simulink model "actuatorsTestHarness"  (R2024a)
settings: configuration reference "standardSILConfiguraitonParams" (kept outside this file)
undefined symbols (not defined in the file): aileronDeflRateLimit_degps, elevatorDeflRateLimit_degps, maxAilDefl_deg, maxElevatorDefl_deg, maxRudderDefl_deg, rudderDeflRateLimit_degps, stepSize_s
settings Model: SimulationMode=accelerator  Creator=jerem  LastModifiedBy=jerem
settings ConfigSetRef: SourceName=standardSILConfiguraitonParams  SourceLocation=Base Workspace

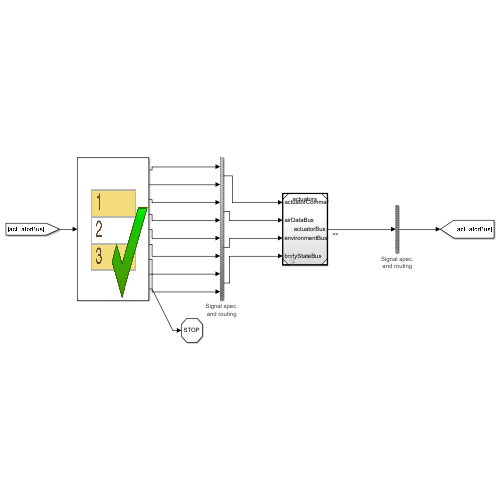
[thumbnail: Simulink's stored preview of the top-level diagram]
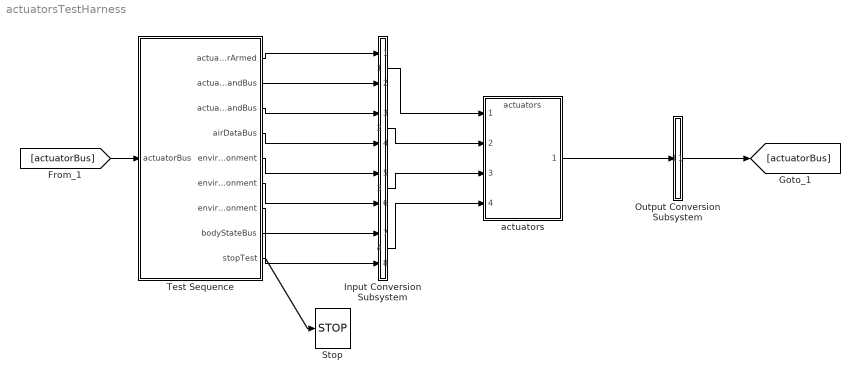
== system actuatorsTestHarness ==
  Input Conversion Subsystem : Subsystem  Tag=__SLT_ICS__  Description=|
      | Signal spec.
      | and routing
      settings: AttributesFormatString=%<Description>
  Output Conversion Subsystem : Subsystem  Tag=__SLT_OCS__  Description=|
      | Signal spec.
      | and routing
      mask init:
      | ICDictionary = get_param(bdroot, 'DataDictionary');
      | if isempty(ICDictionary)
      |    ICScope = Simulink.data.BaseWorkspace;
      | else
      |    ICScope = Simulink.data.DataDictionary(ICDictionary);
      | end
      | 
      | IC1 = Simulink.Bus.createMATLABStruct('ActuatorBus', [], [1 1], ICScope);
      settings: AttributesFormatString=%<Description>
  Stop : Stop
  Test Sequence : Test Sequence  TreatAsAtomicUnit=on
  actuators : ModelReference  ModelNameDialog=actuators  SimulationMode=Normal  ModelReferenceVersion=1.83
  wires:
  Test Sequence/1(actuatorCommandBus_controllerArmed) -> Input Conversion Subsystem/1(Inport_1)
  Test Sequence/2(actuatorCommandBus_ServosCommandBus) -> Input Conversion Subsystem/2(Inport_2)
  Test Sequence/3(actuatorCommandBus_EngineCommandBus) -> Input Conversion Subsystem/3(Inport_3)
  Test Sequence/4(airDataBus) -> Input Conversion Subsystem/4(Inport_4)
  Test Sequence/5(environmentBus_EarthEnvironment) -> Input Conversion Subsystem/5(Inport_5)
  Test Sequence/6(environmentBus_AirEnvironment) -> Input Conversion Subsystem/6(Inport_6)
  Test Sequence/7(environmentBus_TerrainEnvironment) -> Input Conversion Subsystem/7(Inport_7)
  Test Sequence/8(bodyStateBus) -> Input Conversion Subsystem/8(Inport_8)
  [actuatorBus] -> Test Sequence/1(actuatorBus)
  Output Conversion Subsystem/1(Outport_1) -> [actuatorBus]
  Test Sequence/9(stopTest) -> Stop/1
  actuators/1 -> Output Conversion Subsystem/1(Inport_1)
  Input Conversion Subsystem/1(Outport_1) -> actuators/1
  Input Conversion Subsystem/2(Outport_2) -> actuators/2
  Input Conversion Subsystem/3(Outport_3) -> actuators/3
  Input Conversion Subsystem/4(Outport_4) -> actuators/4

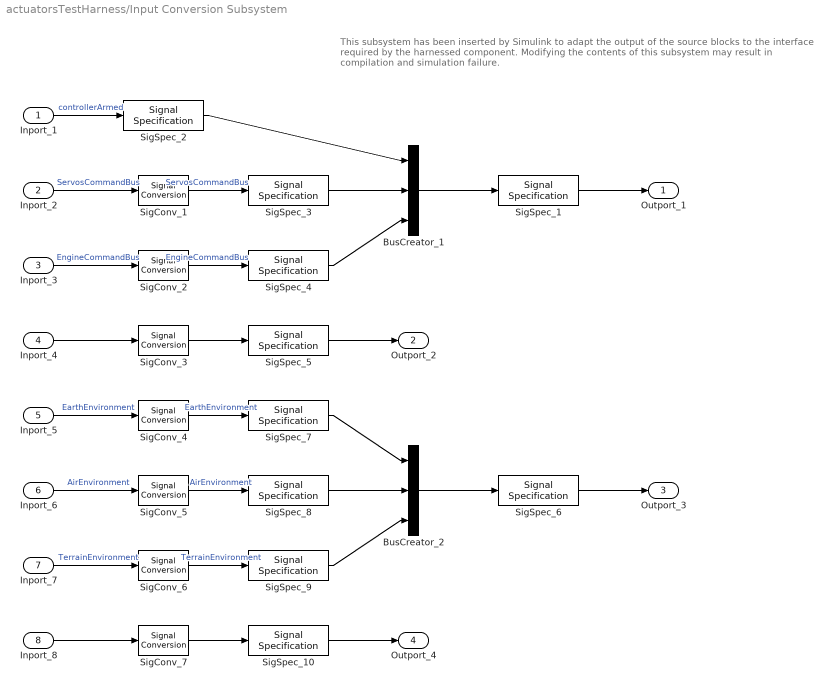
== system actuatorsTestHarness/Input Conversion Subsystem ==
  note: This subsystem has been inserted by Simulink to adapt the output of the source blocks to the interface required by the harnessed component.
      |  Modifying the contents of this subsystem may result in compilation and simulation failure.
  Inport_1 : Inport
  Inport_2 : Inport  Port=2
  Inport_3 : Inport  Port=3
  Inport_4 : Inport  Port=4
  Inport_5 : Inport  Port=5
  Inport_6 : Inport  Port=6
  Inport_7 : Inport  Port=7
  Inport_8 : Inport  Port=8
  BusCreator_1 : BusCreator  Inputs=3  OutDataTypeStr=Bus: ActuatorCommandBus
  BusCreator_2 : BusCreator  Inputs=3  OutDataTypeStr=Bus: EnvironmentBus
  SigConv_{1..2,4..6} (5 alike) : SignalConversion  ConversionOutput=Nonvirtual bus  OverrideOpt=off
  SigConv_3 : SignalConversion  ConversionOutput=Virtual bus  OverrideOpt=off
  SigConv_7 : SignalConversion  ConversionOutput=Virtual bus  OverrideOpt=off
  SigSpec_1 : SignalSpecification  OutDataTypeStr=Bus: ActuatorCommandBus  SampleTime=[-1, 0]
  SigSpec_10 : SignalSpecification  OutDataTypeStr=Bus: BodyStateBus  SampleTime=[-1, 0]
  SigSpec_2 : SignalSpecification  OutDataTypeStr=double  Dimensions=[1]  SampleTime=[-1, 0]
  SigSpec_3 : SignalSpecification  OutDataTypeStr=Bus: ServosCommandBus  Dimensions=[1]  SampleTime=[-1, 0]  BusOutputAsStruct=on
  SigSpec_4 : SignalSpecification  OutDataTypeStr=Bus: EngineCommandBus  Dimensions=[1]  SampleTime=[-1, 0]  BusOutputAsStruct=on
  SigSpec_5 : SignalSpecification  OutDataTypeStr=Bus: AirData  SampleTime=[-1, 0]
  SigSpec_6 : SignalSpecification  OutDataTypeStr=Bus: EnvironmentBus  SampleTime=[-1, 0]
  SigSpec_7 : SignalSpecification  OutDataTypeStr=Bus: EarthEnvironmentBus  Dimensions=[1]  SampleTime=[-1, 0]  BusOutputAsStruct=on
  SigSpec_8 : SignalSpecification  OutDataTypeStr=Bus: AirEnvironmentBus  Dimensions=[1]  SampleTime=[-1, 0]  BusOutputAsStruct=on
  SigSpec_9 : SignalSpecification  OutDataTypeStr=Bus: TerrainEnvironmentBus  Dimensions=[1]  SampleTime=[-1, 0]  BusOutputAsStruct=on
  Outport_1 : Outport
  Outport_2 : Outport  Port=2
  Outport_3 : Outport  Port=3
  Outport_4 : Outport  Port=4
  wires:
  SigSpec_1/1 -> Outport_1/1
  BusCreator_1/1 -> SigSpec_1/1
  SigSpec_2/1 -> BusCreator_1/1
  Inport_1/1 -> SigSpec_2/1  "controllerArmed"
  SigSpec_3/1 -> BusCreator_1/2
  SigConv_1/1 -> SigSpec_3/1  "ServosCommandBus"
  Inport_2/1 -> SigConv_1/1  "ServosCommandBus"
  SigSpec_4/1 -> BusCreator_1/3
  SigConv_2/1 -> SigSpec_4/1  "EngineCommandBus"
  Inport_3/1 -> SigConv_2/1  "EngineCommandBus"
  SigSpec_5/1 -> Outport_2/1
  SigConv_3/1 -> SigSpec_5/1
  Inport_4/1 -> SigConv_3/1
  SigSpec_6/1 -> Outport_3/1
  BusCreator_2/1 -> SigSpec_6/1
  SigSpec_7/1 -> BusCreator_2/1
  SigConv_4/1 -> SigSpec_7/1  "EarthEnvironment"
  Inport_5/1 -> SigConv_4/1  "EarthEnvironment"
  SigSpec_8/1 -> BusCreator_2/2
  SigConv_5/1 -> SigSpec_8/1  "AirEnvironment"
  Inport_6/1 -> SigConv_5/1  "AirEnvironment"
  SigSpec_9/1 -> BusCreator_2/3
  SigConv_6/1 -> SigSpec_9/1  "TerrainEnvironment"
  Inport_7/1 -> SigConv_6/1  "TerrainEnvironment"
  SigSpec_10/1 -> Outport_4/1
  SigConv_7/1 -> SigSpec_10/1
  Inport_8/1 -> SigConv_7/1

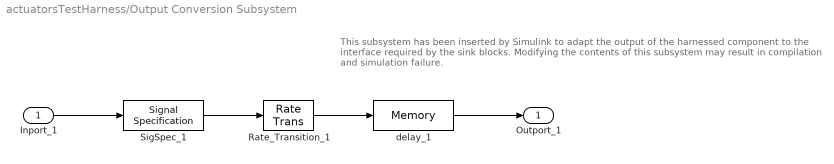
== system actuatorsTestHarness/Output Conversion Subsystem ==
  note: This subsystem has been inserted by Simulink to adapt the output of the harnessed component to the interface required by the sink blocks.
      |  Modifying the contents of this subsystem may result in compilation and simulation failure.
  Inport_1 : Inport
  Rate_Transition_1 : RateTransition  OutPortSampleTimeOpt=Inherit
  SigSpec_1 : SignalSpecification  OutDataTypeStr=Bus: ActuatorBus  Dimensions=[1]
  delay_1 : Memory  InitialCondition=IC1
  Outport_1 : Outport
  wires:
  Inport_1/1 -> SigSpec_1/1
  SigSpec_1/1 -> Rate_Transition_1/1
  Rate_Transition_1/1 -> delay_1/1
  delay_1/1 -> Outport_1/1

== stateflow chart actuatorsTestHarness/Test Sequence ==
  state Scenario_1
    state Initialize
      %% Initialize data outputs.
      actuatorCommandBus_controllerArmed = 0;
      actuatorCommandBus_ServosCommandBus.ServosCommandCustomAircraftBus.cmdControlSurfaceOne_nd = 0;
      actuatorCommandBus_ServosCommandBus.ServosCommandCustomAircraftBus.cmdControlSurfaceTwo_nd = 0;
      actuatorCommandBus_ServosCommandBus.ServosCommandF16Bus.cmdAileron_nd = 0;
      actuatorCommandBus_ServosCommandBus.ServosCommandF16Bus.cmdElevator_nd = 0;
      actuatorCommandBus_ServosCommandBus.ServosCommandF16Bus.cmdRudder_nd = 0;
      actuatorCommandBus_EngineCommandBus.cmdThrottle_unit = 0;
      airDataBus.airspeedInBody_mps = zeros(3,1);
      airDataBus.alpha_rad = 0;
      airDataBus.beta_rad = 0;
      environmentBus_EarthEnvironment.gravityScalar_mps2 = 0;
      environmentBus_EarthEnvironment.worldMagneticFieldInNED_nT = zeros(3,1);
      environmentBus_AirEnvironment.airTemperature_K = 0;
      environmentBus_AirEnvironment.airPressure_Pa = 0;
      environmentBus_AirEnvironment.airDensity_kgpm3 = 0;
      environmentBus_AirEnvironment.windSpeedInNED_mps = zeros(3,1);
      environmentBus_AirEnvironment.speedOfSound_mps = 0;
      environmentBus_AirEnvironment.windsAloftInNED_mps = zeros(3,1);
      environmentBus_AirEnvironment.gustInNED_mps = zeros(3,1);
      environmentBus_AirEnvironment.turbulenceInNED_mps = zeros(3,1);
      environmentBus_TerrainEnvironment.terrainHeightInNED_m = 0;
      bodyStateBus.aircraftVelInNED_mps = zeros(3,1);
      bodyStateBus.aircraftPosInNED_m = zeros(3,1);
      bodyStateBus.aircraftEulerAngles_rad = zeros(3,1);
      bodyStateBus.aircraftVelInBody_mps = zeros(3,1);
      bodyStateBus.aircraftAngVelInBody_radps = zeros(3,1);
      bodyStateBus.aircraftAngAccelInBody_radps2 = zeros(3,1);
      bodyStateBus.aircraftAccelInBody_mps2 = zeros(3,1);
      bodyStateBus.DCM_be = zeros(3,3);
      stopTest = false;
    state verifyControllerDisarmed
      verify(isClose(actuatorBus.EngineBus.angVel_radps, 0))
      verify(isClose(actuatorBus.EngineBus.engineForcesMoments.forcesInBody_N(1), 0))
      verify(isClose(actuatorBus.EngineBus.engineForcesMoments.forcesInBody_N(2), 0))
      verify(isClose(actuatorBus.EngineBus.engineForcesMoments.forcesInBody_N(3), 0))
      verify(isClose(actuatorBus.EngineBus.engineForcesMoments.momentsInBody_Nm(1), 0))
      verify(isClose(actuatorBus.EngineBus.engineForcesMoments.momentsInBody_Nm(2), 0))
      verify(isClose(actuatorBus.EngineBus.engineForcesMoments.momentsInBody_Nm(3), 0))
      verify(isClose(actuatorBus.ServosBus.ServosF16Bus.posAileron_rad,0))
      verify(isClose(actuatorBus.ServosBus.ServosF16Bus.posElevator_rad,0))
      verify(isClose(actuatorBus.ServosBus.ServosF16Bus.posRudder_rad,0))
    state armController
      actuatorCommandBus_controllerArmed = 1;
    state verifyControllerArmed
      verify(isClose(actuatorBus.EngineBus.angVel_radps, 0))
      verify(isClose(actuatorBus.EngineBus.engineForcesMoments.forcesInBody_N(1), 0))
      verify(isClose(actuatorBus.EngineBus.engineForcesMoments.forcesInBody_N(2), 0))
      verify(isClose(actuatorBus.EngineBus.engineForcesMoments.forcesInBody_N(3), 0))
      verify(isClose(actuatorBus.EngineBus.engineForcesMoments.momentsInBody_Nm(1), 0))
      verify(isClose(actuatorBus.EngineBus.engineForcesMoments.momentsInBody_Nm(2), 0))
      verify(isClose(actuatorBus.EngineBus.engineForcesMoments.momentsInBody_Nm(3), 0))
      verify(isClose(actuatorBus.ServosBus.ServosF16Bus.posAileron_rad,0))
      verify(isClose(actuatorBus.ServosBus.ServosF16Bus.posElevator_rad,0))
      verify(isClose(actuatorBus.ServosBus.ServosF16Bus.posRudder_rad,0))
    state maxAileron
      actuatorCommandBus_ServosCommandBus.ServosCommandF16Bus.cmdAileron_nd = 1.1; %This is a normalized value
      previousAileronCmd = actuatorCommandBus_ServosCommandBus.ServosCommandF16Bus.cmdAileron_nd;
    state verifyAileronRate
      aileronCmdRate = (actuatorCommandBus_ServosCommandBus.ServosCommandF16Bus.cmdAileron_nd - previousAileronCmd) * maxAilDefl_deg / stepSize_s;
      verify( aileronCmdRate <= aileronDeflRateLimit_degps)
      previousAileronCmd = actuatorCommandBus_ServosCommandBus.ServosCommandF16Bus.cmdAileron_nd;
    state verifyAileronLimit
      verify(isClose(actuatorBus.ServosBus.ServosF16Bus.posAileron_rad, deg2rad(maxAilDefl_deg)), 'atol', 0.0044) % Tolerance of 0.25 deg used. Arbitrary
    state maxNegAileron
      actuatorCommandBus_ServosCommandBus.ServosCommandF16Bus.cmdAileron_nd = -1.1;
      previousAileronCmd = actuatorCommandBus_ServosCommandBus.ServosCommandF16Bus.cmdAileron_nd;
    state verifyNegAileronRate
      aileronCmdRate = (actuatorCommandBus_ServosCommandBus.ServosCommandF16Bus.cmdAileron_nd - previousAileronCmd) * maxAilDefl_deg / stepSize_s;
      verify( abs(aileronCmdRate) <= aileronDeflRateLimit_degps)
      previousAileronCmd = actuatorCommandBus_ServosCommandBus.ServosCommandF16Bus.cmdAileron_nd;
    state verifyNegAileronLimit
      verify(isClose(actuatorBus.ServosBus.ServosF16Bus.posAileron_rad, -deg2rad(maxAilDefl_deg)), 'atol', 0.0044)
    state maxElevator
      actuatorCommandBus_ServosCommandBus.ServosCommandF16Bus.cmdElevator_nd= 1.1;
      previousElevCmd = actuatorCommandBus_ServosCommandBus.ServosCommandF16Bus.cmdElevator_nd;
    state verifyElevatorRate
      elevatorCmdRate = (actuatorCommandBus_ServosCommandBus.ServosCommandF16Bus.cmdElevator_nd- previousElevCmd ) *maxElevatorDefl_deg / stepSize_s;
      verify( elevatorCmdRate <= elevatorDeflRateLimit_degps)
      previousElevCmd = actuatorCommandBus_ServosCommandBus.ServosCommandF16Bus.cmdElevator_nd;
    state verifyElevatorLimit
      verify(isClose(actuatorBus.ServosBus.ServosF16Bus.posElevator_rad, deg2rad(maxElevatorDefl_deg)), 'atol', 0.0044)
    state maxNegElevator
      actuatorCommandBus_ServosCommandBus.ServosCommandF16Bus.cmdElevator_nd= -1.1;
      previousElevCmd = actuatorCommandBus_ServosCommandBus.ServosCommandF16Bus.cmdElevator_nd;
    state verifyNegElevatorRate
      elevatorCmdRate = (actuatorCommandBus_ServosCommandBus.ServosCommandF16Bus.cmdElevator_nd- previousElevCmd ) * maxElevatorDefl_deg / stepSize_s;
      verify( abs(elevatorCmdRate ) <= elevatorDeflRateLimit_degps)
      previousElevCmd = actuatorCommandBus_ServosCommandBus.ServosCommandF16Bus.cmdElevator_nd;
    state verifyNegElevatorLimit
      verify(isClose(actuatorBus.ServosBus.ServosF16Bus.posElevator_rad, -deg2rad(maxElevatorDefl_deg)), 'atol', 0.0044)
    state maxRudder
      actuatorCommandBus_ServosCommandBus.ServosCommandF16Bus.cmdRudder_nd= 1.1;
      previousRudderCmd = actuatorCommandBus_ServosCommandBus.ServosCommandF16Bus.cmdRudder_nd;
    state verifyRudderRate
      rudderCmdRate = (actuatorCommandBus_ServosCommandBus.ServosCommandF16Bus.cmdRudder_nd - previousRudderCmd) * maxRudderDefl_deg / stepSize_s;
      verify(rudderCmdRate <= rudderDeflRateLimit_degps)
      previousRudderCmd = actuatorCommandBus_ServosCommandBus.ServosCommandF16Bus.cmdRudder_nd;
    state verifyRudderMax
      verify(isClose(actuatorBus.ServosBus.ServosF16Bus.posRudder_rad, deg2rad(maxRudderDefl_deg)), 'atol', 0.0044)
    state maxNegRudder
      actuatorCommandBus_ServosCommandBus.ServosCommandF16Bus.cmdRudder_nd= -1.1;
      previousRudderCmd = actuatorCommandBus_ServosCommandBus.ServosCommandF16Bus.cmdRudder_nd;
    state verifyNegRudderRate
      rudderCmdRate = (actuatorCommandBus_ServosCommandBus.ServosCommandF16Bus.cmdRudder_nd - previousRudderCmd) * maxRudderDefl_deg / stepSize_s;
      verify( abs(rudderCmdRate) <= rudderDeflRateLimit_degps)
      previousRudderCmd = actuatorCommandBus_ServosCommandBus.ServosCommandF16Bus.cmdRudder_nd;
    state verifyNegRudderMax
      verify(isClose(actuatorBus.ServosBus.ServosF16Bus.posRudder_rad, -deg2rad(maxRudderDefl_deg)), 'atol', 0.0044)
    state EndTest
      stopTest = true;
    (default) -> Initialize
    Initialize -> verifyControllerDisarmed : [
        | true
        | ]
    verifyControllerDisarmed -> armController : [
        | after(2,sec)
        | ]
    armController -> verifyControllerArmed : [
        | after(1,sec)
        | ]
    verifyControllerArmed -> maxAileron : [
        | after(1,sec)
        | ]
    maxAileron -> verifyAileronRate : [
        | after(1,tick)
        | ]
    verifyAileronRate -> verifyAileronLimit : [
        | after(1,sec)
        | ]
    verifyAileronLimit -> maxNegAileron : [
        | after(1,sec)
        | ]
    maxNegAileron -> verifyNegAileronRate : [
        | after(1,sec)
        | ]
    verifyNegAileronRate -> verifyNegAileronLimit : [
        | after(1,sec)
        | ]
    verifyNegAileronLimit -> maxElevator : [
        | after(1,sec)
        | ]
    maxElevator -> verifyElevatorRate : [
        | after(1,tick)
        | ]
    verifyElevatorRate -> verifyElevatorLimit : [
        | after(3,sec)
        | ]
    verifyElevatorLimit -> maxNegElevator : [
        | after(1,sec)
        | ]
    maxNegElevator -> verifyNegElevatorRate : [
        | after(1,tick)
        | ]
    verifyNegElevatorRate -> verifyNegElevatorLimit : [
        | after(1,sec)
        | ]
    verifyNegElevatorLimit -> maxRudder : [
        | after(1,sec)
        | ]
    maxRudder -> verifyRudderRate : [
        | after(1,tick)
        | ]
    verifyRudderRate -> verifyRudderMax : [
        | after(1,sec)
        | ]
    verifyRudderMax -> maxNegRudder : [
        | after(1,tick)
        | ]
    maxNegRudder -> verifyNegRudderRate : [
        | after(1,sec)
        | ]
    verifyNegRudderRate -> verifyNegRudderMax : [
        | after(1,sec)
        | ]
    verifyNegRudderMax -> EndTest : [
        | after(1,sec)
        | ]
  (default) -> Scenario_1 : {assert(Active_Scenario_Index == 1,'The value of Scenario Parameter ''Active_Scenario_Index'' is not valid. Use the index of the scenario to specify it.')}
  data: actuatorBus input Bus: ActuatorBus size=[1]; actuatorCommandBus_controllerArmed output double size=[1]; actuatorCommandBus_ServosCommandBus output Bus: ServosCommandBus size=[1]; actuatorCommandBus_EngineCommandBus output Bus: EngineCommandBus size=[1]; airDataBus output Bus: AirData size=[1]; environmentBus_EarthEnvironment output Bus: EarthEnvironmentBus size=[1]; environmentBus_AirEnvironment output Bus: AirEnvironmentBus size=[1]; environmentBus_TerrainEnvironment output Bus: TerrainEnvironmentBus size=[1]; bodyStateBus output Bus: BodyStateBus size=[1]; stopTest output; Active_Scenario_Index parameter =1; maxAilDefl_deg parameter; stepSize_s parameter; aileronDeflRateLimit_degps parameter; previousAileronCmd local; aileronCmdRate local; elevatorDeflRateLimit_degps parameter; maxElevatorDefl_deg parameter; elevatorCmdRate local; previousElevCmd local; rudderDeflRateLimit_degps parameter; maxRudderDefl_deg parameter; previousRudderCmd local; rudderCmdRate local
